simulink library "cctd"  (Simulink 8.1)
settings: Solver=ode1  StartTime=0.0  StopTime=Inf  FixedStep=0.001  RelTol=1e-3
PostLoadFcn:
  | , if any(exist('dsrtsu_mdlpostloadfcn', 'file') == [2, 3, 6]), try dsrtsu_mdlpostloadfcn('Execute', bdroot); catch fprintf('Error in PostLoadFcn (dsrtsu_mdlpostloadfcn) for model "%s":\n %s\n', bdroot, lasterr); end, end,
undefined symbols (not defined in the file or in its folder): C_TICK_TIME_S, ENUM_ACCSTATE_DISABLED, FALSE, KJUD_ACCMaxTimeGap_s, KJUD_ACCMinTimeGap_s, KJUD_ACCTimeGapDelay_ms, TRUE, ZERO_INT
libraries: simulink x1, hcu_lib x1
settings Model: DSRTSU_INTERNAL_RTI_VER=450  DSRTSU_INTERNAL_RTI_TYPE=rti1401  RTICANMMDATA=struct('GeneralSetupData',struct('modelroot','D:\ELN150201_TAIWAN\trunk\AdasDragon\software\sw_development\arch\app\jud','generalsettings',struct('filesettings',struct('destfolder',struct('Name','RTICANMM_FILES','Check',1),'buildfolder',struct('Name','.','Check',1),'AbsDestfolder',struct('Name','D:\ELN150201_TAIWAN\trunk\AdasDragon\software\sw_development\arch\app\jud\RTICANMM_FILES'),'AbsBuildfolder',struct('Name','D:\ELN150201_TAIWAN\trunk\AdasDragon\software\sw_development\arch\app\jud'))),'options',struct('addpaths',1,'rmpaths',1,'addtrcexclusion',logical(1),'cannavigator',struct('checkmonitoring',0),'show_usrtrc',0,'use_usrtrc',0),'advanced',struct('options',[1 1 1 1 1 1 1 1 1 1 1 1 1 1 1 1 1 1 1 1 1 1 1 1 1 1 1 1 1 1 1 1 1 1 1 1 1 1 1 1 1 1 1 1 1 1 1 1 1 1 1 1 1 1 1 1 1 1 1 1 1 1 1 1 1 1 1 1 1 1 1 1 1 1 1 1 1 1 1 1 1 1 1 1 1 1 1 1 1 1 1 1 1 1 1 1 1 1 1 1]),'MPSetup',{{}},'modelname','cctd','block','cctd'))  DSRTSU_INTERNAL_RTIFPGA=40  Creator=AT015411  LastModifiedBy=AT015555

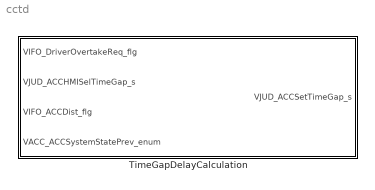
== system cctd ==
  TimeGapDelayCalculation : Subsystem

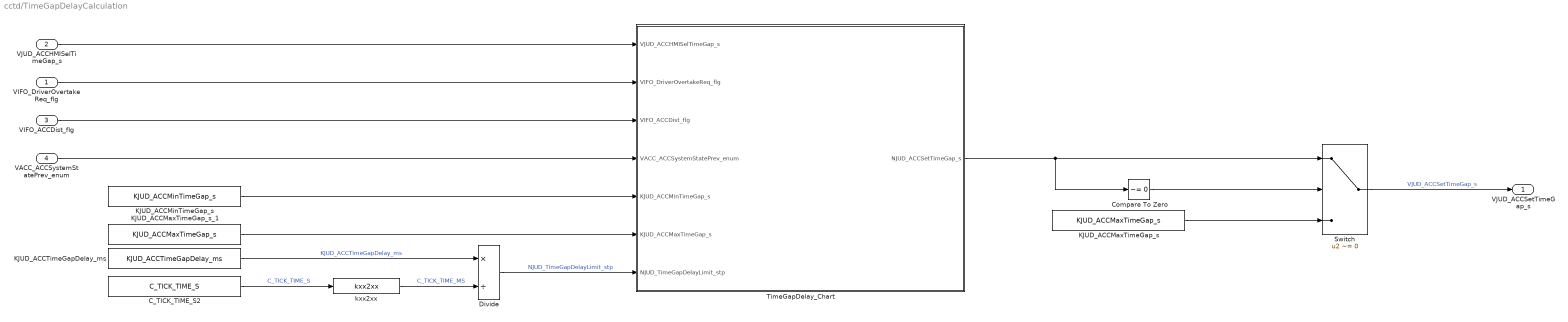
== system cctd/TimeGapDelayCalculation ==
  VIFO_DriverOvertakeReq_flg : Inport
  VJUD_ACCHMISelTimeGap_s : Inport  Port=2
  VIFO_ACCDist_flg : Inport  Port=3
  VACC_ACCSystemStatePrev_enum : Inport  Port=4
  C_TICK_TIME_S2 : Constant  Value=C_TICK_TIME_S  OutDataTypeStr=single
  Compare To Zero : simulink/Logic and Bit Operations/Compare To Zero  relop=~=  OutDataTypeStr=boolean
  Divide : Product  Inputs=*/
  KJUD_ACCMaxTimeGap_s : Constant  Value=KJUD_ACCMaxTimeGap_s  OutDataTypeStr=single
  KJUD_ACCMaxTimeGap_s_1 : Constant  Value=KJUD_ACCMaxTimeGap_s
  KJUD_ACCMinTimeGap_s : Constant  Value=KJUD_ACCMinTimeGap_s
  KJUD_ACCTimeGapDelay_ms : Constant  Value=KJUD_ACCTimeGapDelay_ms  OutDataTypeStr=single
  Switch : Switch  Criteria=u2 ~= 0
  TimeGapDelay_Chart : Stateflow chart  TreatAsAtomicUnit=on
  kxx2xx : hcu_lib/kxx2xx
  VJUD_ACCSetTimeGap_s : Outport
  wires:
  KJUD_ACCMaxTimeGap_s/1 -> Switch/3
  Switch/1 -> VJUD_ACCSetTimeGap_s/1  "VJUD_ACCSetTimeGap_s"
  KJUD_ACCTimeGapDelay_ms/1 -> Divide/1  "KJUD_ACCTimeGapDelay_ms"
  kxx2xx/1 -> Divide/2  "C_TICK_TIME_MS"
  VIFO_ACCDist_flg/1 -> TimeGapDelay_Chart/3(VIFO_ACCDist_flg)
  VJUD_ACCHMISelTimeGap_s/1 -> TimeGapDelay_Chart/1(VJUD_ACCHMISelTimeGap_s)
  Divide/1 -> TimeGapDelay_Chart/7(NJUD_TimeGapDelayLimit_stp)  "NJUD_TimeGapDelayLimit_stp"
  C_TICK_TIME_S2/1 -> kxx2xx/1  "C_TICK_TIME_S"
  TimeGapDelay_Chart/1(NJUD_ACCSetTimeGap_s) -> Compare To Zero/1, Switch/1
  VIFO_DriverOvertakeReq_flg/1 -> TimeGapDelay_Chart/2(VIFO_DriverOvertakeReq_flg)
  VACC_ACCSystemStatePrev_enum/1 -> TimeGapDelay_Chart/4(VACC_ACCSystemStatePrev_enum)
  Compare To Zero/1 -> Switch/2
  KJUD_ACCMinTimeGap_s/1 -> TimeGapDelay_Chart/5(KJUD_ACCMinTimeGap_s)
  KJUD_ACCMaxTimeGap_s_1/1 -> TimeGapDelay_Chart/6(KJUD_ACCMaxTimeGap_s)

== stateflow chart TimeGapDelayCalculation/TimeGapDelay_Chart ==
  state TGAP_CHANGE_ENABLED
    state INITIAL
    state NEW_TGAP
      en:
      NJUD_ACCSetTimeGap_s =VJUD_ACCHMISelTimeGap_s;
    state CHANGING
      state START
        en:
        NJUD_TimeGapDelayLocal_stp = ZERO_INT;
        du:
        NJUD_TimeGapDelayLocal_stp = NJUD_TimeGapDelayLocal_stp+1;
      state RESTART
        en:
        NJUD_TimeGapDelayLocal_stp = ZERO_INT;
      (default) -> START
      START -> RESTART : [VIFO_ACCDist_flg==TRUE]
      RESTART -> START : [VIFO_ACCDist_flg==FALSE]
    state MIN_TGAP
      en:
      NJUD_ACCSetTimeGap_s = KJUD_ACCMinTimeGap_s;
    (default) -> INITIAL
    MIN_TGAP -> NEW_TGAP : [VIFO_DriverOvertakeReq_flg == FALSE]
    INITIAL -> MIN_TGAP [order 2] : [VIFO_DriverOvertakeReq_flg==TRUE...
        | && VIFO_ACCDist_flg==FALSE ]
    CHANGING -> NEW_TGAP : [NJUD_TimeGapDelayLocal_stp >= NJUD_TimeGapDelayLimit_stp]
    INITIAL -> CHANGING [order 1] : [VIFO_ACCDist_flg==TRUE]
    NEW_TGAP -> INITIAL
  state FIRST_VALUE
    en:
    NJUD_ACCSetTimeGap_s=KJUD_ACCMaxTimeGap_s;
  (default) -> FIRST_VALUE
  FIRST_VALUE -> TGAP_CHANGE_ENABLED : [VACC_ACCSystemStatePrev_enum != ENUM_ACCSTATE_DISABLED]
  TGAP_CHANGE_ENABLED -> FIRST_VALUE : [VACC_ACCSystemStatePrev_enum == ENUM_ACCSTATE_DISABLED]
  data: VJUD_ACCHMISelTimeGap_s input double; VIFO_DriverOvertakeReq_flg input double; VIFO_ACCDist_flg input double; VACC_ACCSystemStatePrev_enum input double; KJUD_ACCMinTimeGap_s input double; KJUD_ACCMaxTimeGap_s input double; NJUD_ACCSetTimeGap_s output single; NJUD_TimeGapDelayLimit_stp input double; NJUD_TimeGapDelayLocal_stp local single; TRUE parameter boolean; FALSE parameter boolean; ZERO_INT parameter int8; ENUM_ACCSTATE_DISABLED parameter uint8
